simulink model "Osc"  (R2020b)
settings: Solver=FixedStepDiscrete  StartTime=0.0  StopTime=1000.0  FixedStep=1  RelTol=1e-3
settings Model: Creator=ncleju  LastModifiedBy=ncleju

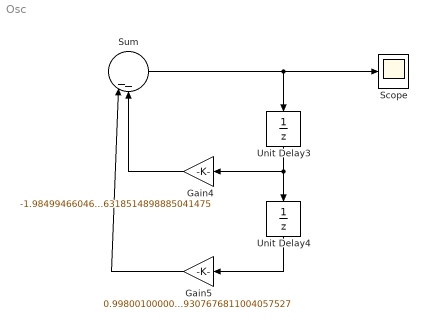
== system Osc ==
  Gain4 : Gain  Gain=-1.984994660460841275906318514898885041475
  Gain5 : Gain  Gain=0.998001000000000026979307676811004057527
  Scope : Scope
  Sum : Sum  Inputs=|||||--
  Unit Delay3 : UnitDelay  InitialCondition=1  SampleTime=-1  HasFrameUpgradeWarning=on
  Unit Delay4 : UnitDelay  SampleTime=-1  HasFrameUpgradeWarning=on
  wires:
  Sum/1 -> Scope/1, Unit Delay3/1
  Unit Delay3/1 -> Gain4/1, Unit Delay4/1
  Unit Delay4/1 -> Gain5/1
  Gain4/1 -> Sum/2
  Gain5/1 -> Sum/1
